simulink model "relative_distance_tracking"  (R2018b)
settings: Solver=FixedStepAuto  StartTime=0.0  StopTime=40  FixedStep=0.05  RelTol=1e-3
settings Model: Creator=suvo.ganguli  LastModifiedBy=suvo.ganguli

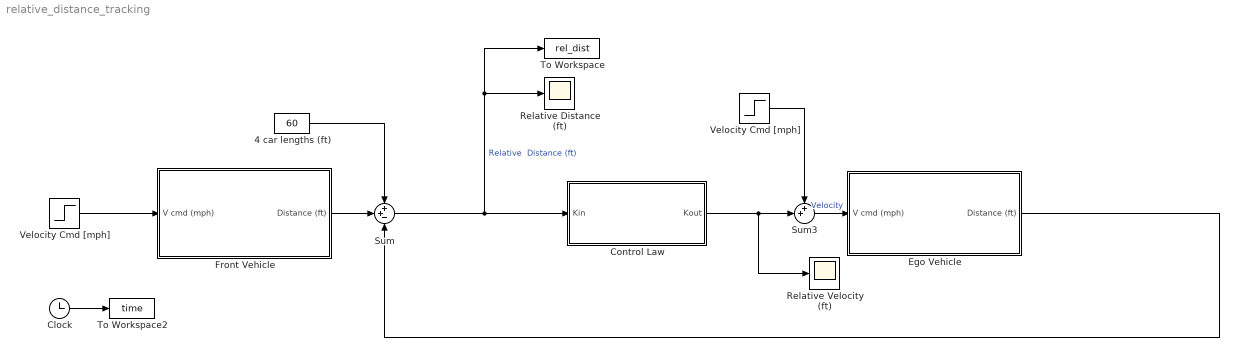
== system relative_distance_tracking ==
  4 car lengths (ft) : Constant  Value=60
  Clock : Clock
  Control Law : Subsystem
  Ego Vehicle : Subsystem
  Front Vehicle : Subsystem
  Relative Distance (ft) : Scope
  Relative Velocity (ft) : Scope
  Sum : Sum  Inputs=++-
  Sum3 : Sum  Inputs=++|
  To Workspace : ToWorkspace  VariableName=rel_dist  SaveFormat=Timeseries  SampleTime=-1
  To Workspace2 : ToWorkspace  VariableName=time  SampleTime=-1
  Velocity Cmd [mph] : Step  Before=45  After=55  SampleTime=0
  "Velocity Cmd [mph] " : Step  Before=45  After=45  SampleTime=0
  wires:
  Clock/1 -> To Workspace2/1
  Velocity Cmd [mph]/1 -> Front Vehicle/1(V cmd (mph))
  "Velocity Cmd [mph] "/1 -> Sum3/1
  Sum3/1 -> Ego Vehicle/1(V cmd (mph))  "Velocity"
  Sum/1 -> Control Law/1(Kin), To Workspace/1, Relative Distance (ft)/1  "Relative  Distance (ft)"
  Front Vehicle/1(Distance (ft)) -> Sum/2
  Ego Vehicle/1(Distance (ft)) -> Sum/3
  4 car lengths (ft)/1 -> Sum/1
  Control Law/1(Kout) -> Relative Velocity (ft)/1, Sum3/2

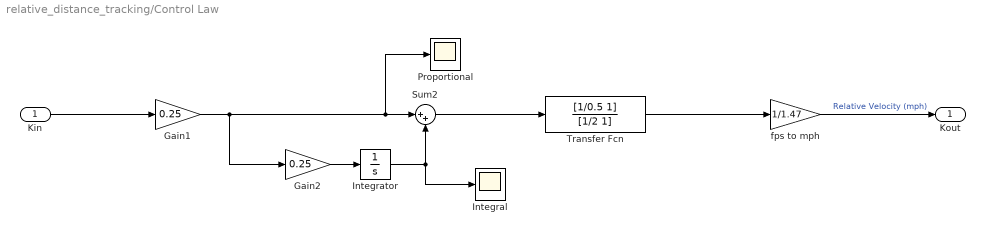
== system relative_distance_tracking/Control Law ==
  Kin : Inport
  Gain1 : Gain  Gain=0.25
  Gain2 : Gain  Gain=0.25
  Integral : Scope
  Integrator : Integrator
  Proportional : Scope
  Sum2 : Sum  Inputs=|++
  Transfer Fcn : TransferFcn  Numerator=[1/0.5 1]  Denominator=[1/2 1]
  fps to mph : Gain  Gain=1/1.47
  Kout : Outport
  wires:
  Gain2/1 -> Integrator/1
  Integrator/1 -> Sum2/2, Integral/1
  Sum2/1 -> Transfer Fcn/1
  Gain1/1 -> Gain2/1, Proportional/1, Sum2/1
  fps to mph/1 -> Kout/1  "Relative Velocity (mph)"
  Kin/1 -> Gain1/1
  Transfer Fcn/1 -> fps to mph/1

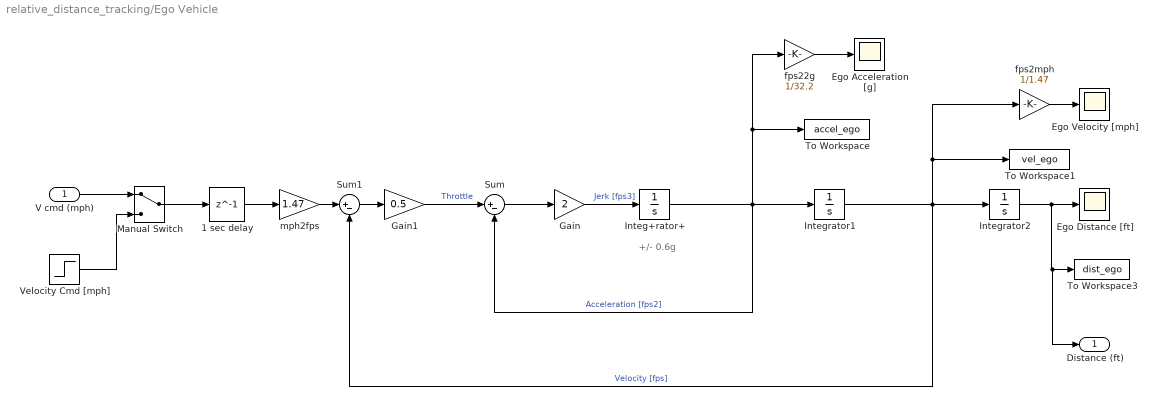
== system relative_distance_tracking/Ego Vehicle ==
  note: +/- 0.6g
  V cmd (mph) : Inport
  1 sec delay : Delay  DelayLength=1  InitialCondition=45
  Ego Acceleration [g] : Scope
  Ego Distance [ft] : Scope
  Ego Velocity [mph] : Scope
  Gain : Gain  Gain=2
  Gain1 : Gain  Gain=0.5
  Integ+rator+ : Integrator  LimitOutput=on  UpperSaturationLimit=0.6*32.2  LowerSaturationLimit=-0.6*32.2
  Integrator1 : Integrator  InitialCondition=45*1.47
  Integrator2 : Integrator
  Manual Switch : ManualSwitch
  Sum : Sum  Inputs=|+-
  Sum1 : Sum  Inputs=|+-
  To Workspace : ToWorkspace  VariableName=accel_ego  SampleTime=-1
  To Workspace1 : ToWorkspace  VariableName=vel_ego  SampleTime=-1
  To Workspace3 : ToWorkspace  VariableName=dist_ego  SampleTime=-1
  Velocity Cmd [mph] : Step  Time=0  Before=20  After=0  SampleTime=0
  fps22g : Gain  Gain=1/32.2
  fps2mph : Gain  Gain=1/1.47
  mph2fps : Gain  Gain=1.47
  Distance (ft) : Outport
  wires:
  Gain/1 -> Integ+rator+/1  "Jerk [fps3]"
  fps2mph/1 -> Ego Velocity [mph]/1
  Integrator1/1 -> Sum1/2, Integrator2/1, To Workspace1/1, fps2mph/1  "Velocity [fps]"
  Sum/1 -> Gain/1
  Integ+rator+/1 -> Integrator1/1, To Workspace/1, fps22g/1, Sum/2  "Acceleration [fps2]"
  Sum1/1 -> Gain1/1
  1 sec delay/1 -> mph2fps/1
  Integrator2/1 -> Distance (ft)/1, To Workspace3/1, Ego Distance [ft]/1
  fps22g/1 -> Ego Acceleration [g]/1
  mph2fps/1 -> Sum1/1
  Gain1/1 -> Sum/1  "Throttle"
  Manual Switch/1 -> 1 sec delay/1
  Velocity Cmd [mph]/1 -> Manual Switch/2
  V cmd (mph)/1 -> Manual Switch/1

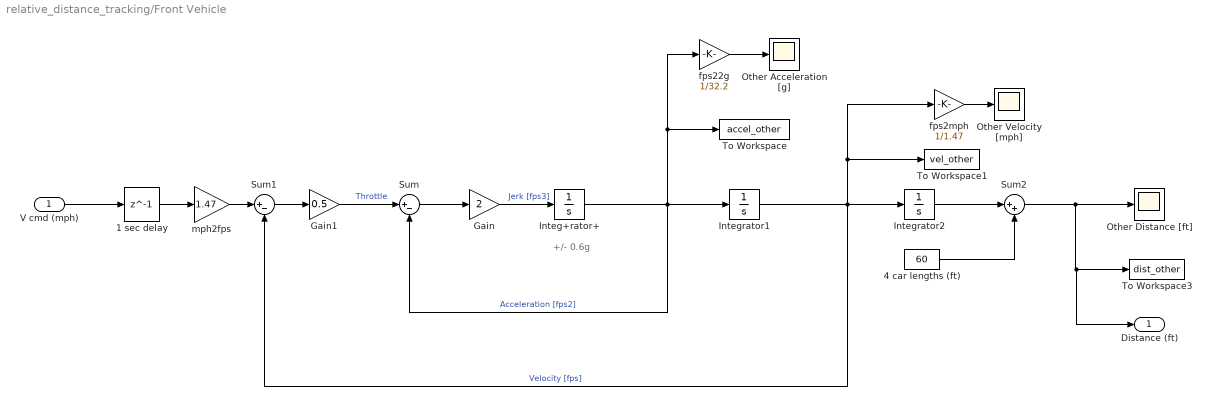
== system relative_distance_tracking/Front Vehicle ==
  note: +/- 0.6g
  V cmd (mph) : Inport
  1 sec delay : Delay  DelayLength=1  InitialCondition=45
  4 car lengths (ft) : Constant  Value=60
  Gain : Gain  Gain=2
  Gain1 : Gain  Gain=0.5
  Integ+rator+ : Integrator  LimitOutput=on  UpperSaturationLimit=0.6*32.2  LowerSaturationLimit=-0.6*32.2
  Integrator1 : Integrator  InitialCondition=45*1.47
  Integrator2 : Integrator
  Other Acceleration [g] : Scope
  Other Distance [ft] : Scope
  Other Velocity [mph] : Scope
  Sum : Sum  Inputs=|+-
  Sum1 : Sum  Inputs=|+-
  Sum2 : Sum  Inputs=|++
  To Workspace : ToWorkspace  VariableName=accel_other  SampleTime=-1
  To Workspace1 : ToWorkspace  VariableName=vel_other  SampleTime=-1
  To Workspace3 : ToWorkspace  VariableName=dist_other  SampleTime=-1
  fps22g : Gain  Gain=1/32.2
  fps2mph : Gain  Gain=1/1.47
  mph2fps : Gain  Gain=1.47
  Distance (ft) : Outport
  wires:
  Gain1/1 -> Sum/1  "Throttle"
  mph2fps/1 -> Sum1/1
  fps22g/1 -> Other Acceleration [g]/1
  V cmd (mph)/1 -> 1 sec delay/1
  1 sec delay/1 -> mph2fps/1
  Sum1/1 -> Gain1/1
  Integ+rator+/1 -> Sum/2, fps22g/1, To Workspace/1, Integrator1/1  "Acceleration [fps2]"
  Sum/1 -> Gain/1
  Integrator1/1 -> fps2mph/1, To Workspace1/1, Integrator2/1, Sum1/2  "Velocity [fps]"
  fps2mph/1 -> Other Velocity [mph]/1
  Gain/1 -> Integ+rator+/1  "Jerk [fps3]"
  Integrator2/1 -> Sum2/1
  Sum2/1 -> Distance (ft)/1, To Workspace3/1, Other Distance [ft]/1
  4 car lengths (ft)/1 -> Sum2/2
